simulink model "dvig_2"  (Simulink 8.9)
settings: Solver=ode45  StartTime=0.0  StopTime=2  MaxStep=0.01  MinStep=0.0001  RelTol=1e-3  AbsTol=1e-3  EnableMultiTasking=on
settings Model: Creator=ras19  LastModifiedBy=ras19
settings DataIOCC: SaveOutput=off  SaveTime=off  SignalLoggingName=sigsOut
settings OptimizationCC: LifeSpan=auto
settings DebuggingCC: SaveWithParameterizedLinksMsg=none  SignalResolutionControl=TryResolveAllWithWarning  MultiTaskDSMMsg=warning  MultiTaskCondExecSysMsg=none  FcnCallInpInsideContextMsg=error  StateNameClashWarn=none  SFUnexpectedBacktrackingDiag=error  SFNoUnconditionalDefaultTransitionDiag=error  SFExecutionAtInitializationDiag=warning
settings HardwareCC: TargetUnknown=on
settings GRTTargetCC: GeneratePreprocessorConditionals=Use local settings

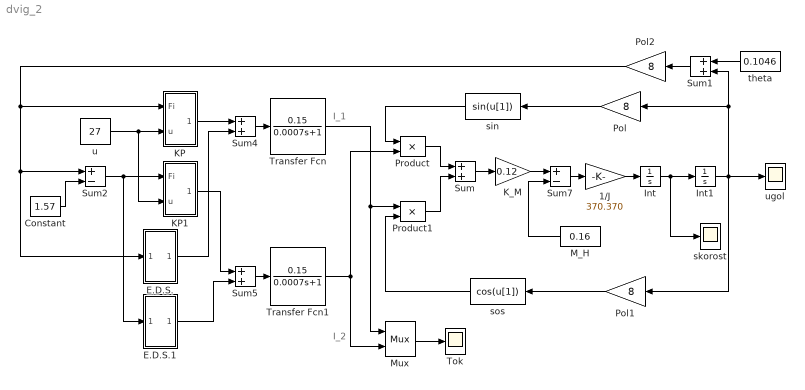
== system dvig_2 ==
  note: I_1
  note: I_2
  1/J : Gain  Gain=370.370  SaturateOnIntegerOverflow=on  OutDataTypeStr=Inherit: Same as input  ParamDataTypeStr=Inherit: Same as input
  Constant : Constant  Value=1.57
  E.D.S. : Subsystem
  E.D.S.1 : Subsystem
  Int : Integrator
  Int1 : Integrator
  KP : Subsystem
  KP1 : Subsystem
  K_M : Gain  Gain=0.12  SaturateOnIntegerOverflow=on  OutDataTypeStr=Inherit: Same as input  ParamDataTypeStr=Inherit: Same as input
  M_H : Constant  Value=0.16
  Mux : Mux  Inputs=2
  Pol : Gain  Gain=8  SaturateOnIntegerOverflow=on  OutDataTypeStr=Inherit: Same as input  ParamDataTypeStr=Inherit: Same as input
  Pol1 : Gain  Gain=8  SaturateOnIntegerOverflow=on  OutDataTypeStr=Inherit: Same as input  ParamDataTypeStr=Inherit: Same as input
  Pol2 : Gain  Gain=8  SaturateOnIntegerOverflow=on  OutDataTypeStr=Inherit: Same as input  ParamDataTypeStr=Inherit: Same as input
  Product : Product  SaturateOnIntegerOverflow=on  InputSameDT=on  OutDataTypeStr=Inherit: Same as first input
  Product1 : Product  SaturateOnIntegerOverflow=on  InputSameDT=on  OutDataTypeStr=Inherit: Same as first input
  Sum{,1,4..5} (4 alike) : Sum  SaturateOnIntegerOverflow=on  InputSameDT=on  OutDataTypeStr=Inherit: Same as first input
  Sum2 : Sum  Inputs=+-  SaturateOnIntegerOverflow=on  InputSameDT=on  OutDataTypeStr=Inherit: Same as first input
  Sum7 : Sum  Inputs=+-  SaturateOnIntegerOverflow=on  InputSameDT=on  OutDataTypeStr=Inherit: Same as first input
  Tok : Scope
  Transfer Fcn : TransferFcn  Numerator=[0.15]  Denominator=[0.0007 1]
  Transfer Fcn1 : TransferFcn  Numerator=[0.15]  Denominator=[0.0007 1]
  sin : Fcn
  skorost : Scope
  sos : Fcn  Expr=cos(u[1])
  theta : Constant  Value=0.1046
  u : Constant  Value=27
  ugol : Scope
  wires:
  Sum/1 -> K_M/1
  1/J/1 -> Int/1
  Int/1 -> Int1/1, skorost/1
  Pol/1 -> sin/1
  Pol1/1 -> sos/1
  sin/1 -> Product/1
  sos/1 -> Product1/2
  theta/1 -> Sum1/1
  Int1/1 -> Sum1/2, Pol/1, Pol1/1, ugol/1
  Sum1/1 -> Pol2/1
  Constant/1 -> Sum2/2
  u/1 -> KP/2(u), KP1/2(u)
  Pol2/1 -> KP/1(Fi), Sum2/1, E.D.S./1(in_1)
  Sum4/1 -> Transfer Fcn/1
  KP/1(out_1) -> Sum4/1
  Sum5/1 -> Transfer Fcn1/1
  KP1/1(out_1) -> Sum5/1
  E.D.S./1(out_1) -> Sum4/2
  E.D.S.1/1(out_1) -> Sum5/2
  Product/1 -> Sum/1
  Product1/1 -> Sum/2
  Sum7/1 -> 1/J/1
  M_H/1 -> Sum7/2
  Sum2/1 -> E.D.S.1/1(in_1), KP1/1(Fi)
  Transfer Fcn/1 -> Product1/1, Mux/1
  Mux/1 -> Tok/1
  K_M/1 -> Sum7/1
  Transfer Fcn1/1 -> Product/2, Mux/2

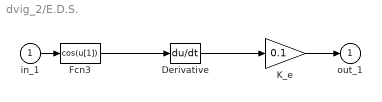
== system dvig_2/E.D.S. ==
  in_1 : Inport
  Derivative : Derivative
  Fcn3 : Fcn  Expr=cos(u[1])
  K_e : Gain  Gain=0.1  SaturateOnIntegerOverflow=on  OutDataTypeStr=Inherit: Same as input  ParamDataTypeStr=Inherit: Same as input
  out_1 : Outport
  wires:
  Fcn3/1 -> Derivative/1
  in_1/1 -> Fcn3/1
  Derivative/1 -> K_e/1
  K_e/1 -> out_1/1

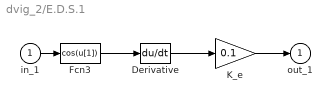
== system dvig_2/E.D.S.1 ==
  in_1 : Inport
  Derivative : Derivative
  Fcn3 : Fcn  Expr=cos(u[1])
  K_e : Gain  Gain=0.1  SaturateOnIntegerOverflow=on  OutDataTypeStr=Inherit: Same as input  ParamDataTypeStr=Inherit: Same as input
  out_1 : Outport
  wires:
  Derivative/1 -> K_e/1
  in_1/1 -> Fcn3/1
  Fcn3/1 -> Derivative/1
  K_e/1 -> out_1/1

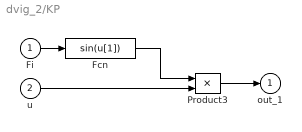
== system dvig_2/KP ==
  Fi : Inport
  u : Inport  Port=2
  Fcn : Fcn
  Product3 : Product  SaturateOnIntegerOverflow=on  InputSameDT=on  OutDataTypeStr=Inherit: Same as first input
  out_1 : Outport
  wires:
  Fi/1 -> Fcn/1
  Product3/1 -> out_1/1
  u/1 -> Product3/2
  Fcn/1 -> Product3/1

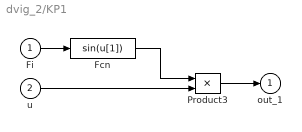
== system dvig_2/KP1 ==
  Fi : Inport
  u : Inport  Port=2
  Fcn : Fcn
  Product3 : Product  SaturateOnIntegerOverflow=on  InputSameDT=on  OutDataTypeStr=Inherit: Same as first input
  out_1 : Outport
  wires:
  Fcn/1 -> Product3/1
  u/1 -> Product3/2
  Product3/1 -> out_1/1
  Fi/1 -> Fcn/1
